simulink model "regolatore_spazio_operativo"  (R2024b)
settings: Solver=VariableStepAuto  StartTime=0.0  StopTime=100  RelTol=1e-3
values from neighbouring files (symbols this model uses):
  kd = K(:,3:4)    [regolatore_robot.m]
  kp = K(:,1:2)    [regolatore_robot.m]
settings Model: Creator=Davide  LastModifiedBy=david
settings OptimizationCC: ReuseModelBlockBuffer=off
settings RTWCC: GPUComputeCapability=3.5

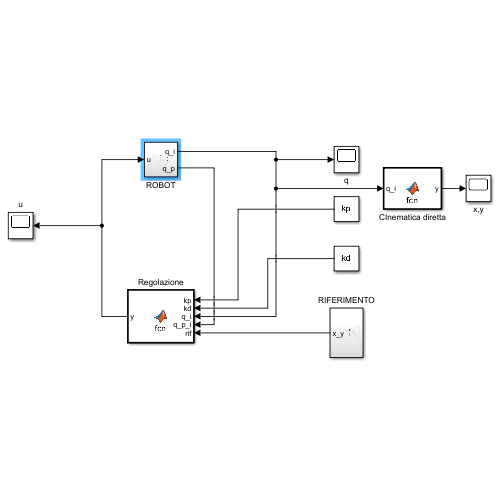
[thumbnail: Simulink's stored preview of the top-level diagram]
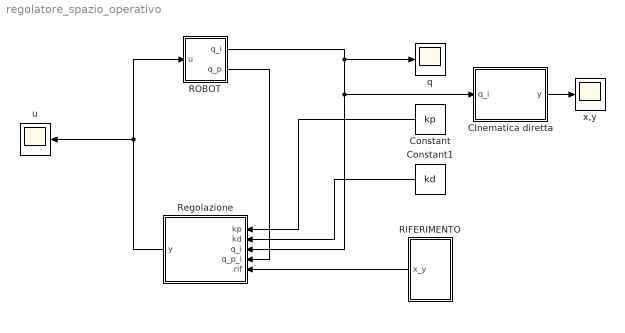
== system regolatore_spazio_operativo ==
  CInematica diretta : MATLAB Function  TreatAsAtomicUnit=on
  Constant : Constant  Value=kp  VectorParams1D=off
  Constant1 : Constant  Value=kd  VectorParams1D=off
  RIFERIMENTO : Subsystem
  ROBOT : Subsystem
  Regolazione : MATLAB Function  TreatAsAtomicUnit=on
  q : Scope
  u : Scope
  x,y : Scope
  wires:
  Regolazione/1(y) -> u/1, ROBOT/1(u)
  ROBOT/1(q_i) -> q/1, CInematica diretta/1(q_i), Regolazione/3(q_i)
  ROBOT/2(q_p) -> Regolazione/4(q_p_i)
  Constant/1 -> Regolazione/1(kp)
  Constant1/1 -> Regolazione/2(kd)
  CInematica diretta/1(y) -> x,y/1
  RIFERIMENTO/1(x_y) -> Regolazione/5(rif)

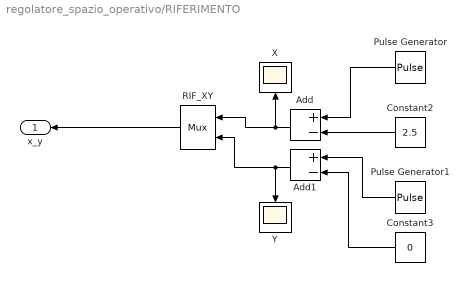
== system regolatore_spazio_operativo/RIFERIMENTO ==
  Add : Sum  Inputs=+-
  Add1 : Sum  Inputs=+-
  Constant2 : Constant  Value=2.5  VectorParams1D=off
  Constant3 : Constant  Value=0  VectorParams1D=off
  Pulse Generator : DiscretePulseGenerator  PulseType=Time based  Amplitude=3.5  Period=10  PulseWidth=50  VectorParams1D=off
  Pulse Generator1 : DiscretePulseGenerator  PulseType=Time based  Period=10  PulseWidth=50  VectorParams1D=off
  RIF_XY : Mux  Inputs=2
      settings: DisplayOption=signals
  X : Scope
  Y : Scope
  x_y : Outport
  wires:
  Add1/1 -> Y/1, RIF_XY/2
  Pulse Generator1/1 -> Add1/1
  Constant3/1 -> Add1/2
  Pulse Generator/1 -> Add/1
  Constant2/1 -> Add/2
  Add/1 -> RIF_XY/1, X/1
  RIF_XY/1 -> x_y/1

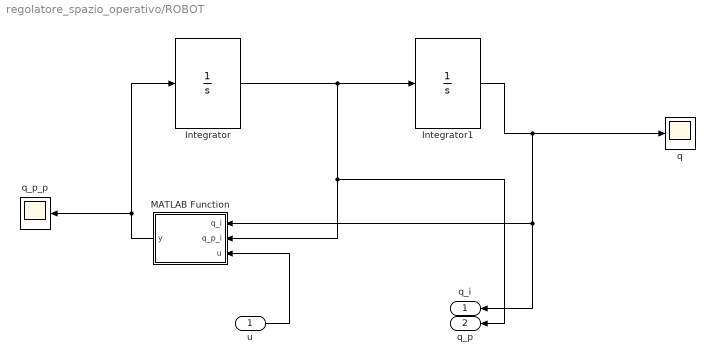
== system regolatore_spazio_operativo/ROBOT ==
  u : Inport
  Integrator : Integrator  InitialCondition=[0;0]
  Integrator1 : Integrator  InitialCondition=[0;0]
  MATLAB Function : MATLAB Function  TreatAsAtomicUnit=on
  q : Scope
  q_p_p : Scope
  q_i : Outport
  q_p : Outport  Port=2
  wires:
  u/1 -> MATLAB Function/3(u)
  Integrator/1 -> q_p/1, MATLAB Function/2(q_p_i), Integrator1/1
  MATLAB Function/1(y) -> Integrator/1, q_p_p/1
  Integrator1/1 -> q_i/1, MATLAB Function/1(q_i), q/1

== matlab function regolatore_spazio_operativo/ROBOT/MATLAB Function ==
  data: q_i input; q_p_i input; u input; y output
function y = fcn(q_i,q_p_i,u)


theta1 = 10.6125; 
theta2 = 0.85; 
theta3 = 2.25;
theta4 = 1.6;
theta5 = 80.9325;
theta6 = 14.7150;
q = q_i;
q_p = q_p_i;
v = u;
F1 = 15;
F2 = 10;

B = [theta1 + 2*theta3*q(2) theta2+theta3*cos(q(2)) ; ...
     theta2+theta3*cos(q(2)) theta4];
C = [-2*theta3*q_p(2)*sin(q(2))  -theta3*q_p(2)*sin(q(2)) ; ...
      theta3*q_p(1)*sin(q(2))              0              ];
g = [theta5*cos(q(1))+theta6*cos(q(1)+q(2)) ; theta6*cos(q(1)+q(2))];
F = [F1*q_p(1) ; F2*q_p(2)];

y = inv(B)*(v - g - F - C*q_p);

== matlab function regolatore_spazio_operativo/Regolazione ==
  data: kp input; kd input; q_i input; q_p_i input; rif input; y output
function y = fcn(kp,kd,q_i,q_p_i,rif)


l1 = 1.5;
l2 = 1;

theta5 = 80.9325;
theta6 = 14.7150;
q = q_i;
q_p = q_p_i;
r = rif;
f = [l1*cos(q(1))+l2*cos(q(1)+q(2)) ; l1*sin(q(1))+l2*sin(q(1)+q(2))];

g = [theta5*cos(q(1))+theta6*cos(q(1)+q(2)) ; theta6*cos(q(1)+q(2))];
J = [- sin(q(1) + q(2)) - (3*sin(q(1)))/2 -sin(q(1) + q(2)) ;
      cos(q(1) + q(2)) + (3*cos(q(1)))/2  cos(q(1) + q(2))  ];

y = g + J' *kp*(r-f) - kd*q_p;

== matlab function regolatore_spazio_operativo/CInematica diretta ==
  data: q_i input; y output
function y = fcn(q_i)

q = q_i;
l1 = 1.5;
l2 = 1;

%Estrazione posizione spazio operativo
y = [l1*cos(q(1))+l2*cos(q(1)+q(2)) ; l1*sin(q(1))+l2*sin(q(1)+q(2))];
